simulink model "VCU_CS75_12_27_test"  (R2014a)
settings: Solver=FixedStepDiscrete  StartTime=0.0  StopTime=25  FixedStep=0.0005  RelTol=1e-3
undefined symbols (not defined in the file): D1, D2, D3, ecucoder_acal, ErrorSumMax1, ErrorSumMax2, ErrorSumMax3, I1, I2, I3, I_SW01_L, LaterlAngleCommand, LDW, P1, P2, P3, RemoteAcclPosition
libraries: simulink x913, ec5744lib x39
(part 12 of 30)

== system VCU_CS75_12_27_test/长安CS75底盘程序，20ms一次/Output/Subsystem/TransmitMessages5/ACC_3F5 ==
  ACC_AEBTargetLngRange_in : Inport
  ACC_AEBTargetRelSpeed_in : Inport  Port=2
  ACC_AEBTargetLatRange_in : Inport  Port=3
  ACC_HostPotentialTargetLatRng_in : Inport  Port=4
  ACC_HostPotentialTargetDetection_in : Inport  Port=5
  ACC_HostPotentialTargetLngRng_in : Inport  Port=6
  RollingConter_in : Inport  Port=7
  ACC_HostPotentialTargetType_in : Inport  Port=8
  CRC_in : Inport  Port=9
  ACC_3F5_DLC : Constant  Value=8  OutDataTypeStr=uint8
  ACC_3F5_DLC_Out : Terminator
  ACC_3F5_ID : Constant  Value=1013  OutDataTypeStr=single
  ACC_3F5_ID_Out : Terminator
  ACC_3F5_mux : Mux  Inputs=8
  ACC_AEBTargetLatRange : Subsystem
  ACC_AEBTargetLngRange : Subsystem
  ACC_AEBTargetRelSpeed : Subsystem
  ACC_HostPotentialTargetDetection : Subsystem
  ACC_HostPotentialTargetLatRng : Subsystem
  ACC_HostPotentialTargetLngRng : Subsystem
  ACC_HostPotentialTargetType : Subsystem
  CRC : Subsystem
  Conv{1..8} (8 alike) : DataTypeConversion
  RollingConter : Subsystem
  or{1..8} (8 alike) : simulink/Logic and Bit Operations/Bitwise Operator  logicop=OR  UseBitMask=off  NumInputPorts=9  BitMask=bin2dec('11011001')  BitMaskRealWorld=Stored Integer
  output : Outport
  wires:
  ACC_3F5_mux/1 -> output/1
  ACC_AEBTargetLngRange/1(output1) -> or1/1
  ACC_AEBTargetLngRange/2(output2) -> or2/1
  ACC_AEBTargetLngRange/3(output3) -> or3/1
  ACC_AEBTargetLngRange/4(output4) -> or4/1
  ACC_AEBTargetLngRange/5(output5) -> or5/1
  ACC_AEBTargetLngRange/6(output6) -> or6/1
  ACC_AEBTargetLngRange/7(output7) -> or7/1
  ACC_AEBTargetLngRange/8(output8) -> or8/1
  ACC_AEBTargetRelSpeed/1(output1) -> or1/2
  ACC_AEBTargetRelSpeed/2(output2) -> or2/2
  ACC_AEBTargetRelSpeed/3(output3) -> or3/2
  ACC_AEBTargetRelSpeed/4(output4) -> or4/2
  ACC_AEBTargetRelSpeed/5(output5) -> or5/2
  ACC_AEBTargetRelSpeed/6(output6) -> or6/2
  ACC_AEBTargetRelSpeed/7(output7) -> or7/2
  ACC_AEBTargetRelSpeed/8(output8) -> or8/2
  ACC_AEBTargetLatRange/1(output1) -> or1/3
  ACC_AEBTargetLatRange/2(output2) -> or2/3
  ACC_AEBTargetLatRange/3(output3) -> or3/3
  ACC_AEBTargetLatRange/4(output4) -> or4/3
  ACC_AEBTargetLatRange/5(output5) -> or5/3
  ACC_AEBTargetLatRange/6(output6) -> or6/3
  ACC_AEBTargetLatRange/7(output7) -> or7/3
  ACC_AEBTargetLatRange/8(output8) -> or8/3
  ACC_HostPotentialTargetLatRng/1(output1) -> or1/4
  ACC_HostPotentialTargetLatRng/2(output2) -> or2/4
  ACC_HostPotentialTargetLatRng/3(output3) -> or3/4
  ACC_HostPotentialTargetLatRng/4(output4) -> or4/4
  ACC_HostPotentialTargetLatRng/5(output5) -> or5/4
  ACC_HostPotentialTargetLatRng/6(output6) -> or6/4
  ACC_HostPotentialTargetLatRng/7(output7) -> or7/4
  ACC_HostPotentialTargetLatRng/8(output8) -> or8/4
  ACC_HostPotentialTargetDetection/1(output1) -> or1/5
  ACC_HostPotentialTargetDetection/2(output2) -> or2/5
  ACC_HostPotentialTargetDetection/3(output3) -> or3/5
  ACC_HostPotentialTargetDetection/4(output4) -> or4/5
  ACC_HostPotentialTargetDetection/5(output5) -> or5/5
  ACC_HostPotentialTargetDetection/6(output6) -> or6/5
  ACC_HostPotentialTargetDetection/7(output7) -> or7/5
  ACC_HostPotentialTargetDetection/8(output8) -> or8/5
  ACC_HostPotentialTargetLngRng/1(output1) -> or1/6
  ACC_HostPotentialTargetLngRng/2(output2) -> or2/6
  ACC_HostPotentialTargetLngRng/3(output3) -> or3/6
  ACC_HostPotentialTargetLngRng/4(output4) -> or4/6
  ACC_HostPotentialTargetLngRng/5(output5) -> or5/6
  ACC_HostPotentialTargetLngRng/6(output6) -> or6/6
  ACC_HostPotentialTargetLngRng/7(output7) -> or7/6
  ACC_HostPotentialTargetLngRng/8(output8) -> or8/6
  RollingConter/1(output1) -> or1/7
  RollingConter/2(output2) -> or2/7
  RollingConter/3(output3) -> or3/7
  RollingConter/4(output4) -> or4/7
  RollingConter/5(output5) -> or5/7
  RollingConter/6(output6) -> or6/7
  RollingConter/7(output7) -> or7/7
  RollingConter/8(output8) -> or8/7
  ACC_HostPotentialTargetType/1(output1) -> or1/8
  ACC_HostPotentialTargetType/2(output2) -> or2/8
  ACC_HostPotentialTargetType/3(output3) -> or3/8
  ACC_HostPotentialTargetType/4(output4) -> or4/8
  ACC_HostPotentialTargetType/5(output5) -> or5/8
  ACC_HostPotentialTargetType/6(output6) -> or6/8
  ACC_HostPotentialTargetType/7(output7) -> or7/8
  ACC_HostPotentialTargetType/8(output8) -> or8/8
  CRC/1(output1) -> or1/9
  CRC/2(output2) -> or2/9
  CRC/3(output3) -> or3/9
  CRC/4(output4) -> or4/9
  CRC/5(output5) -> or5/9
  CRC/6(output6) -> or6/9
  CRC/7(output7) -> or7/9
  CRC/8(output8) -> or8/9
  or1/1 -> Conv1/1
  Conv1/1 -> ACC_3F5_mux/1
  or2/1 -> Conv2/1
  Conv2/1 -> ACC_3F5_mux/2
  or3/1 -> Conv3/1
  Conv3/1 -> ACC_3F5_mux/3
  or4/1 -> Conv4/1
  Conv4/1 -> ACC_3F5_mux/4
  or5/1 -> Conv5/1
  Conv5/1 -> ACC_3F5_mux/5
  or6/1 -> Conv6/1
  Conv6/1 -> ACC_3F5_mux/6
  or7/1 -> Conv7/1
  Conv7/1 -> ACC_3F5_mux/7
  or8/1 -> Conv8/1
  Conv8/1 -> ACC_3F5_mux/8
  ACC_3F5_ID/1 -> ACC_3F5_ID_Out/1
  ACC_3F5_DLC/1 -> ACC_3F5_DLC_Out/1
  ACC_AEBTargetLngRange_in/1 -> ACC_AEBTargetLngRange/1(ACC_AEBTargetLngRange)
  ACC_AEBTargetRelSpeed_in/1 -> ACC_AEBTargetRelSpeed/1(ACC_AEBTargetRelSpeed)
  ACC_AEBTargetLatRange_in/1 -> ACC_AEBTargetLatRange/1(ACC_AEBTargetLatRange)
  ACC_HostPotentialTargetLatRng_in/1 -> ACC_HostPotentialTargetLatRng/1(ACC_HostPotentialTargetLatRng)
  ACC_HostPotentialTargetDetection_in/1 -> ACC_HostPotentialTargetDetection/1(ACC_HostPotentialTargetDetection)
  ACC_HostPotentialTargetLngRng_in/1 -> ACC_HostPotentialTargetLngRng/1(ACC_HostPotentialTargetLngRng)
  RollingConter_in/1 -> RollingConter/1(RollingConter)
  ACC_HostPotentialTargetType_in/1 -> ACC_HostPotentialTargetType/1(ACC_HostPotentialTargetType)
  CRC_in/1 -> CRC/1(CRC)

== system VCU_CS75_12_27_test/长安CS75底盘程序，20ms一次/Output/Subsystem/TransmitMessages7/APA_29A ==
  APA_EPBrequest_in : Inport
  APA_EPBrequestValid_in : Inport  Port=2
  APA_TranShiftReqValid_in : Inport  Port=3
  APA_TranShiftRequest_in : Inport  Port=4
  APA_TargetAcceleration_in : Inport  Port=5
  APA_TargetAccelerationValid_in : Inport  Port=6
  APA_GearReqValid_in : Inport  Port=7
  APA_LSCAction_in : Inport  Port=8
  APA_ActivationStatus_in : Inport  Port=9
  APA_RollingCounter_in : Inport  Port=10
  APA_Checksum_in : Inport  Port=11
  APA_29A_DLC : Constant  Value=8  OutDataTypeStr=uint8
  APA_29A_DLC_Out : Terminator
  APA_29A_ID : Constant  Value=666  OutDataTypeStr=single
  APA_29A_ID_Out : Terminator
  APA_29A_mux : Mux  Inputs=8
  APA_ActivationStatus : Subsystem
  APA_Checksum : Subsystem
  APA_EPBrequest : Subsystem
  APA_EPBrequestValid : Subsystem
  APA_GearReqValid : Subsystem
  APA_LSCAction : Subsystem
  APA_RollingCounter : Subsystem
  APA_TargetAcceleration : Subsystem
  APA_TargetAccelerationValid : Subsystem
  APA_TranShiftReqValid : Subsystem
  APA_TranShiftRequest : Subsystem
  Conv{1..8} (8 alike) : DataTypeConversion
  or{1..8} (8 alike) : simulink/Logic and Bit Operations/Bitwise Operator  logicop=OR  UseBitMask=off  NumInputPorts=11  BitMask=bin2dec('11011001')  BitMaskRealWorld=Stored Integer
  output : Outport
  wires:
  APA_29A_mux/1 -> output/1
  APA_EPBrequest/1(output1) -> or1/1
  APA_EPBrequest/2(output2) -> or2/1
  APA_EPBrequest/3(output3) -> or3/1
  APA_EPBrequest/4(output4) -> or4/1
  APA_EPBrequest/5(output5) -> or5/1
  APA_EPBrequest/6(output6) -> or6/1
  APA_EPBrequest/7(output7) -> or7/1
  APA_EPBrequest/8(output8) -> or8/1
  APA_EPBrequestValid/1(output1) -> or1/2
  APA_EPBrequestValid/2(output2) -> or2/2
  APA_EPBrequestValid/3(output3) -> or3/2
  APA_EPBrequestValid/4(output4) -> or4/2
  APA_EPBrequestValid/5(output5) -> or5/2
  APA_EPBrequestValid/6(output6) -> or6/2
  APA_EPBrequestValid/7(output7) -> or7/2
  APA_EPBrequestValid/8(output8) -> or8/2
  APA_TranShiftReqValid/1(output1) -> or1/3
  APA_TranShiftReqValid/2(output2) -> or2/3
  APA_TranShiftReqValid/3(output3) -> or3/3
  APA_TranShiftReqValid/4(output4) -> or4/3
  APA_TranShiftReqValid/5(output5) -> or5/3
  APA_TranShiftReqValid/6(output6) -> or6/3
  APA_TranShiftReqValid/7(output7) -> or7/3
  APA_TranShiftReqValid/8(output8) -> or8/3
  APA_TranShiftRequest/1(output1) -> or1/4
  APA_TranShiftRequest/2(output2) -> or2/4
  APA_TranShiftRequest/3(output3) -> or3/4
  APA_TranShiftRequest/4(output4) -> or4/4
  APA_TranShiftRequest/5(output5) -> or5/4
  APA_TranShiftRequest/6(output6) -> or6/4
  APA_TranShiftRequest/7(output7) -> or7/4
  APA_TranShiftRequest/8(output8) -> or8/4
  APA_TargetAcceleration/1(output1) -> or1/5
  APA_TargetAcceleration/2(output2) -> or2/5
  APA_TargetAcceleration/3(output3) -> or3/5
  APA_TargetAcceleration/4(output4) -> or4/5
  APA_TargetAcceleration/5(output5) -> or5/5
  APA_TargetAcceleration/6(output6) -> or6/5
  APA_TargetAcceleration/7(output7) -> or7/5
  APA_TargetAcceleration/8(output8) -> or8/5
  APA_TargetAccelerationValid/1(output1) -> or1/6
  APA_TargetAccelerationValid/2(output2) -> or2/6
  APA_TargetAccelerationValid/3(output3) -> or3/6
  APA_TargetAccelerationValid/4(output4) -> or4/6
  APA_TargetAccelerationValid/5(output5) -> or5/6
  APA_TargetAccelerationValid/6(output6) -> or6/6
  APA_TargetAccelerationValid/7(output7) -> or7/6
  APA_TargetAccelerationValid/8(output8) -> or8/6
  APA_GearReqValid/1(output1) -> or1/7
  APA_GearReqValid/2(output2) -> or2/7
  APA_GearReqValid/3(output3) -> or3/7
  APA_GearReqValid/4(output4) -> or4/7
  APA_GearReqValid/5(output5) -> or5/7
  APA_GearReqValid/6(output6) -> or6/7
  APA_GearReqValid/7(output7) -> or7/7
  APA_GearReqValid/8(output8) -> or8/7
  APA_LSCAction/1(output1) -> or1/8
  APA_LSCAction/2(output2) -> or2/8
  APA_LSCAction/3(output3) -> or3/8
  APA_LSCAction/4(output4) -> or4/8
  APA_LSCAction/5(output5) -> or5/8
  APA_LSCAction/6(output6) -> or6/8
  APA_LSCAction/7(output7) -> or7/8
  APA_LSCAction/8(output8) -> or8/8
  APA_ActivationStatus/1(output1) -> or1/9
  APA_ActivationStatus/2(output2) -> or2/9
  APA_ActivationStatus/3(output3) -> or3/9
  APA_ActivationStatus/4(output4) -> or4/9
  APA_ActivationStatus/5(output5) -> or5/9
  APA_ActivationStatus/6(output6) -> or6/9
  APA_ActivationStatus/7(output7) -> or7/9
  APA_ActivationStatus/8(output8) -> or8/9
  APA_RollingCounter/1(output1) -> or1/10
  APA_RollingCounter/2(output2) -> or2/10
  APA_RollingCounter/3(output3) -> or3/10
  APA_RollingCounter/4(output4) -> or4/10
  APA_RollingCounter/5(output5) -> or5/10
  APA_RollingCounter/6(output6) -> or6/10
  APA_RollingCounter/7(output7) -> or7/10
  APA_RollingCounter/8(output8) -> or8/10
  APA_Checksum/1(output1) -> or1/11
  APA_Checksum/2(output2) -> or2/11
  APA_Checksum/3(output3) -> or3/11
  APA_Checksum/4(output4) -> or4/11
  APA_Checksum/5(output5) -> or5/11
  APA_Checksum/6(output6) -> or6/11
  APA_Checksum/7(output7) -> or7/11
  APA_Checksum/8(output8) -> or8/11
  or1/1 -> Conv1/1
  Conv1/1 -> APA_29A_mux/1
  or2/1 -> Conv2/1
  Conv2/1 -> APA_29A_mux/2
  or3/1 -> Conv3/1
  Conv3/1 -> APA_29A_mux/3
  or4/1 -> Conv4/1
  Conv4/1 -> APA_29A_mux/4
  or5/1 -> Conv5/1
  Conv5/1 -> APA_29A_mux/5
  or6/1 -> Conv6/1
  Conv6/1 -> APA_29A_mux/6
  or7/1 -> Conv7/1
  Conv7/1 -> APA_29A_mux/7
  or8/1 -> Conv8/1
  Conv8/1 -> APA_29A_mux/8
  APA_29A_ID/1 -> APA_29A_ID_Out/1
  APA_29A_DLC/1 -> APA_29A_DLC_Out/1
  APA_EPBrequest_in/1 -> APA_EPBrequest/1(APA_EPBrequest)
  APA_EPBrequestValid_in/1 -> APA_EPBrequestValid/1(APA_EPBrequestValid)
  APA_TranShiftReqValid_in/1 -> APA_TranShiftReqValid/1(APA_TranShiftReqValid)
  APA_TranShiftRequest_in/1 -> APA_TranShiftRequest/1(APA_TranShiftRequest)
  APA_TargetAcceleration_in/1 -> APA_TargetAcceleration/1(APA_TargetAcceleration)
  APA_TargetAccelerationValid_in/1 -> APA_TargetAccelerationValid/1(APA_TargetAccelerationValid)
  APA_GearReqValid_in/1 -> APA_GearReqValid/1(APA_GearReqValid)
  APA_LSCAction_in/1 -> APA_LSCAction/1(APA_LSCAction)
  APA_ActivationStatus_in/1 -> APA_ActivationStatus/1(APA_ActivationStatus)
  APA_RollingCounter_in/1 -> APA_RollingCounter/1(APA_RollingCounter)
  APA_Checksum_in/1 -> APA_Checksum/1(APA_Checksum)

== system VCU_CS75_12_27_test/长安CS75底盘程序，20ms一次/Output/Subsystem/TransmitMessages8/APA_2D4 ==
  APA_APAStatus_in : Inport
  APA_ReleasePressureReq_in : Inport  Port=2
  RollingConter_in : Inport  Port=3
  CRC_in : Inport  Port=4
  APA_2D4_DLC : Constant  Value=8  OutDataTypeStr=uint8
  APA_2D4_DLC_Out : Terminator
  APA_2D4_ID : Constant  Value=724  OutDataTypeStr=single
  APA_2D4_ID_Out : Terminator
  APA_2D4_mux : Mux  Inputs=8
  APA_APAStatus : Subsystem
  APA_ReleasePressureReq : Subsystem
  CRC : Subsystem
  Conv{1..8} (8 alike) : DataTypeConversion
  RollingConter : Subsystem
  or{1..8} (8 alike) : simulink/Logic and Bit Operations/Bitwise Operator  logicop=OR  UseBitMask=off  NumInputPorts=4  BitMask=bin2dec('11011001')  BitMaskRealWorld=Stored Integer
  output : Outport
  wires:
  APA_2D4_mux/1 -> output/1
  APA_APAStatus/1(output1) -> or1/1
  APA_APAStatus/2(output2) -> or2/1
  APA_APAStatus/3(output3) -> or3/1
  APA_APAStatus/4(output4) -> or4/1
  APA_APAStatus/5(output5) -> or5/1
  APA_APAStatus/6(output6) -> or6/1
  APA_APAStatus/7(output7) -> or7/1
  APA_APAStatus/8(output8) -> or8/1
  APA_ReleasePressureReq/1(output1) -> or1/2
  APA_ReleasePressureReq/2(output2) -> or2/2
  APA_ReleasePressureReq/3(output3) -> or3/2
  APA_ReleasePressureReq/4(output4) -> or4/2
  APA_ReleasePressureReq/5(output5) -> or5/2
  APA_ReleasePressureReq/6(output6) -> or6/2
  APA_ReleasePressureReq/7(output7) -> or7/2
  APA_ReleasePressureReq/8(output8) -> or8/2
  RollingConter/1(output1) -> or1/3
  RollingConter/2(output2) -> or2/3
  RollingConter/3(output3) -> or3/3
  RollingConter/4(output4) -> or4/3
  RollingConter/5(output5) -> or5/3
  RollingConter/6(output6) -> or6/3
  RollingConter/7(output7) -> or7/3
  RollingConter/8(output8) -> or8/3
  CRC/1(output1) -> or1/4
  CRC/2(output2) -> or2/4
  CRC/3(output3) -> or3/4
  CRC/4(output4) -> or4/4
  CRC/5(output5) -> or5/4
  CRC/6(output6) -> or6/4
  CRC/7(output7) -> or7/4
  CRC/8(output8) -> or8/4
  or1/1 -> Conv1/1
  Conv1/1 -> APA_2D4_mux/1
  or2/1 -> Conv2/1
  Conv2/1 -> APA_2D4_mux/2
  or3/1 -> Conv3/1
  Conv3/1 -> APA_2D4_mux/3
  or4/1 -> Conv4/1
  Conv4/1 -> APA_2D4_mux/4
  or5/1 -> Conv5/1
  Conv5/1 -> APA_2D4_mux/5
  or6/1 -> Conv6/1
  Conv6/1 -> APA_2D4_mux/6
  or7/1 -> Conv7/1
  Conv7/1 -> APA_2D4_mux/7
  or8/1 -> Conv8/1
  Conv8/1 -> APA_2D4_mux/8
  APA_2D4_ID/1 -> APA_2D4_ID_Out/1
  APA_2D4_DLC/1 -> APA_2D4_DLC_Out/1
  APA_APAStatus_in/1 -> APA_APAStatus/1(APA_APAStatus)
  APA_ReleasePressureReq_in/1 -> APA_ReleasePressureReq/1(APA_ReleasePressureReq)
  RollingConter_in/1 -> RollingConter/1(RollingConter)
  CRC_in/1 -> CRC/1(CRC)

== system VCU_CS75_12_27_test/长安CS75底盘程序，20ms一次/Input/CAN0_Rx/a1_211/ReceiveMessages/Subsystem ==
  note: -5~100
  note: -100~100
  input : Inport
  Enable : EnablePort
  Bus Creator : BusCreator  Inputs=5
  Constant : Constant  Value=0  SampleTime=-1
  Constant1 : Constant  Value=0  SampleTime=-1
  Constant2 : Constant  Value=0  SampleTime=-1
  Data Store Write : DataStoreWrite  DataStoreName=Vx_out  DataStoreElements=Vx_out
  Data Store Write1 : DataStoreWrite  DataStoreName=mission_out  DataStoreElements=mission_out
  Data Store Write2 : DataStoreWrite  DataStoreName=SCS_out  DataStoreElements=SCS_out
  Data Store Write3 : DataStoreWrite  DataStoreName=finish_out  DataStoreElements=finish_out
  Data Store Write4 : DataStoreWrite  DataStoreName=tap_out  DataStoreElements=tap_out
  Data Store Write5 : DataStoreWrite  DataStoreName=cones_count_all_out  DataStoreElements=cones_count_all_out
  Data Store Write6 : DataStoreWrite  DataStoreName=cones_count_actual_out  DataStoreElements=cones_count_actual_out
  Data Type Conversion : DataTypeConversion  OutDataTypeStr=double
  MATLAB Function1 : MATLAB Function  TreatAsAtomicUnit=on
  Signal Conversion : SignalConversion
  a1 : Subsystem
  A1_211 : Outport
  wires:
  MATLAB Function1/1(y) -> Bus Creator/2  "RemoteAcclPosition"
  Constant/1 -> Bus Creator/4  "A1_Message_Counter"
  Constant1/1 -> Bus Creator/5  "A1_Checksum"
  input/1 -> a1/1(input)
  Constant2/1 -> Bus Creator/1  "AutoDrivingReady"
  a1/8(throttlevbrake_position_Out) -> Data Type Conversion/1  "RemoteAcclPosition"
  a1/1(Vx_Out) -> Data Store Write/1
  a1/2(mission_Out) -> Data Store Write1/1
  a1/3(SCS_Out) -> Data Store Write2/1
  a1/4(finish_Out) -> Data Store Write3/1
  a1/5(tap_Out) -> Data Store Write4/1
  a1/6(cones_count_all_Out) -> Data Store Write5/1
  a1/7(cones_count_actual_Out) -> Data Store Write6/1
  Bus Creator/1 -> Signal Conversion/1
  Data Type Conversion/1 -> MATLAB Function1/1(u)
  Signal Conversion/1 -> A1_211/1
  a1/9(target_steering_Out) -> Bus Creator/3  "LaterlAngleCommand"

== system VCU_CS75_12_27_test/长安CS75底盘程序，20ms一次/Input/CAN1_Rx/BCM_288/ReceiveMessages/Subsystem ==
  input : Inport
  Enable : EnablePort
  BCM_1 : Subsystem
  Bus Creator : BusCreator  Inputs=20
  Signal Conversion : SignalConversion
  BCM_288 : Outport
  wires:
  Bus Creator/1 -> Signal Conversion/1
  input/1 -> BCM_1/1(input)
  BCM_1/1(BCM_FrontWashStatus_Out) -> Bus Creator/1  "BCM_FrontWashStatus"
  BCM_1/2(BCM_TurnIndicatorRight_Out) -> Bus Creator/2  "BCM_TurnIndicatorRight"
  BCM_1/3(BCM_TurnIndicatorLeft_Out) -> Bus Creator/3  "BCM_TurnIndicatorLeft"
  BCM_1/4(BCM_HoodStatus_Out) -> Bus Creator/4  "BCM_HoodStatus"
  BCM_1/5(BCM_TrunkDoorStatus_Out) -> Bus Creator/5  "BCM_TrunkDoorStatus"
  BCM_1/6(BCM_RightRearDoorStatus_Out) -> Bus Creator/6  "BCM_RightRearDoorStatus"
  BCM_1/7(BCM_LeftRearDoorStatus_Out) -> Bus Creator/7  "BCM_LeftRearDoorStatus"
  BCM_1/8(BCM_PassengerDoorStatus_Out) -> Bus Creator/8  "BCM_PassengerDoorStatus"
  BCM_1/9(BCM_DriverDoorStatus_Out) -> Bus Creator/9  "BCM_DriverDoorStatus"
  BCM_1/10(BCM_PassengerDoorLockStatus_Out) -> Bus Creator/10  "BCM_PassengerDoorLockStatus"
  BCM_1/11(BCM_emergencylightstatus_Out) -> Bus Creator/11  "BCM_emergencylightstatus"
  BCM_1/12(BCM_DriverDoorLockStatus_Out) -> Bus Creator/12  "BCM_DriverDoorLockStatus"
  BCM_1/13(BCM_PowerStatusFeedback_Out) -> Bus Creator/13  "BCM_PowerStatusFeedback"
  BCM_1/14(BCM_RearWiperStatus_Out) -> Bus Creator/14  "BCM_RearWiperStatus"
  BCM_1/15(BCM_FrontWiperStatus_Out) -> Bus Creator/15  "BCM_FrontWiperStatus"
  BCM_1/16(BCM_ReversePosition_Out) -> Bus Creator/16  "BCM_ReversePosition"
  BCM_1/17(BCM_TurnLightSwitchSts_Out) -> Bus Creator/17  "BCM_TurnLightSwitchSts"
  BCM_1/18(BCM_BuzzerWarningMode_Out) -> Bus Creator/18  "BCM_BuzzerWarningMode"
  BCM_1/19(BCM_SystemFailureFlag_Out) -> Bus Creator/19  "BCM_SystemFailureFlag"
  BCM_1/20(BCM_LatchOverheatProtect_Out) -> Bus Creator/20  "BCM_LatchOverheatProtect"
  Signal Conversion/1 -> BCM_288/1

== system VCU_CS75_12_27_test/长安CS75底盘程序，20ms一次/Input/CAN1_Rx/BCM_328/ReceiveMessages/Subsystem ==
  input : Inport
  Enable : EnablePort
  BCM_1 : Subsystem
  Bus Creator : BusCreator  Inputs=6
  Signal Conversion : SignalConversion
  BCM_328 : Outport
  wires:
  Bus Creator/1 -> Signal Conversion/1
  input/1 -> BCM_1/1(input)
  BCM_1/1(LCM_DriveMode_Out) -> Bus Creator/1  "LCM_DriveMode"
  BCM_1/2(LCM_DRLSts_Out) -> Bus Creator/2  "LCM_DRLSts"
  BCM_1/3(LCM_LASSwitch_Out) -> Bus Creator/3  "LCM_LASSwitch"
  BCM_1/4(LCM_RearRightTuningLightFaultSts_Out) -> Bus Creator/4  "LCM_RearRightTuningLightFaultSts"
  BCM_1/5(LCM_RearLeftTuningLightFaultSts_Out) -> Bus Creator/5  "LCM_RearLeftTuningLightFaultSts"
  BCM_1/6(LCM_ReverseLightSts_Out) -> Bus Creator/6  "LCM_ReverseLightSts"
  Signal Conversion/1 -> BCM_328/1

== system VCU_CS75_12_27_test/长安CS75底盘程序，20ms一次/Input/CAN1_Rx/BCM_348/ReceiveMessages/Subsystem ==
  input : Inport
  Enable : EnablePort
  BCM_1 : Subsystem
  Bus Creator : BusCreator  Inputs=3
  Signal Conversion : SignalConversion
  BCM_348 : Outport
  wires:
  input/1 -> BCM_1/1(input)
  Bus Creator/1 -> Signal Conversion/1
  BCM_1/1(BCM_DriveMode_Out) -> Bus Creator/1  "BCM_DriveMode"
  BCM_1/2(BCM_LockSignal_Out) -> Bus Creator/2  "BCM_LockSignal"
  BCM_1/3(BCM_UnlockSignal_Out) -> Bus Creator/3  "BCM_UnlockSignal"
  Signal Conversion/1 -> BCM_348/1

== system VCU_CS75_12_27_test/长安CS75底盘程序，20ms一次/Input/CAN1_Rx/BCM_3DF/ReceiveMessages/Subsystem ==
  input : Inport
  Enable : EnablePort
  BCM_3DF1 : Subsystem
  Bus Creator : BusCreator  Inputs=8
  Signal Conversion : SignalConversion
  BCM_3DF : Outport
  wires:
  Bus Creator/1 -> Signal Conversion/1
  input/1 -> BCM_3DF1/1(input)
  BCM_3DF1/1(BCM_DriveMode_Out) -> Bus Creator/1  "BCM_DriveMode"
  BCM_3DF1/2(BCM_EPSTorqueMode_Out) -> Bus Creator/2  "BCM_EPSTorqueMode"
  BCM_3DF1/3(BCM_DriveModeStatus_Out) -> Bus Creator/3  "BCM_DriveModeStatus"
  BCM_3DF1/4(BCM_DriveModeFeedback_Out) -> Bus Creator/4  "BCM_DriveModeFeedback"
  BCM_3DF1/5(BCM_EPSTorqueModeFeedback_Out) -> Bus Creator/5  "BCM_EPSTorqueModeFeedback"
  BCM_3DF1/6(BCM_AmbientLightColorFeedback_Out) -> Bus Creator/6  "BCM_AmbientLightColorFeedback"
  BCM_3DF1/7(BCM_RollingCounter_Out) -> Bus Creator/7  "BCM_RollingCounter"
  BCM_3DF1/8(BCM_CRC_Checksum_Out) -> Bus Creator/8  "BCM_CRC_Checksum"
  Signal Conversion/1 -> BCM_3DF/1

== system VCU_CS75_12_27_test/长安CS75底盘程序，20ms一次/Input/CAN1_Rx/EMS_205/ReceiveMessages/Subsystem ==
  input : Inport
  Enable : EnablePort
  Bus Creator : BusCreator  Inputs=7
  EMS : Subsystem
  Signal Conversion : SignalConversion
  EMS_205 : Outport
  wires:
  EMS/1(EMS_ESPTorqReuestAvailability_Out) -> Bus Creator/1  "EMS_ESPTorqReuestAvailability"
  EMS/2(EMS_TorqFailure_Out) -> Bus Creator/2  "EMS_TorqFailure"
  EMS/3(EMS_IndicatedDriverReqTorq_Out) -> Bus Creator/3  "EMS_IndicatedDriverReqTorq"
  EMS/4(EMS_FrictionalTorq_Out) -> Bus Creator/4  "EMS_FrictionalTorq"
  EMS/5(EMS_IndicatedRealEngTorq_Out) -> Bus Creator/5  "EMS_IndicatedRealEngTorq"
  EMS/6(EMS_RollingCounter_id205_Out) -> Bus Creator/6  "EMS_RollingCounter_id205"
  EMS/7(EMS_CheckSum_205_Out) -> Bus Creator/7  "EMS_CheckSum_205"
  input/1 -> EMS/1(input)
  Bus Creator/1 -> Signal Conversion/1
  Signal Conversion/1 -> EMS_205/1

== system VCU_CS75_12_27_test/长安CS75底盘程序，20ms一次/Input/CAN1_Rx/EMS_255/ReceiveMessages/Subsystem ==
  input : Inport
  Enable : EnablePort
  Bus Creator : BusCreator  Inputs=7
  EMS : Subsystem
  Signal Conversion : SignalConversion
  EMS_255 : Outport
  wires:
  input/1 -> EMS/1(input)
  Bus Creator/1 -> Signal Conversion/1
  EMS/1(EMS_BrakePedalStatus_Out) -> Bus Creator/1  "EMS_BrakePedalStatus"
  EMS/2(EMS_AccpedelError_Out) -> Bus Creator/2  "EMS_AccpedelError"
  EMS/3(EMS_EngineSpeedError_Out) -> Bus Creator/3  "EMS_EngineSpeedError"
  EMS/4(EMS_EngineSpeed_Out) -> Bus Creator/4  "EMS_EngineSpeed"
  EMS/5(EMS_AccPedal_Out) -> Bus Creator/5  "EMS_AccPedal"
  EMS/6(EMS_RollingCounter_id255_Out) -> Bus Creator/6  "EMS_RollingCounter_id255"
  EMS/7(EMS_CheckSum_255_Out) -> Bus Creator/7  "EMS_CheckSum_255"
  Signal Conversion/1 -> EMS_255/1

== system VCU_CS75_12_27_test/长安CS75底盘程序，20ms一次/Input/CAN1_Rx/EMS_265/ReceiveMessages/Subsystem ==
  input : Inport
  Enable : EnablePort
  Bus Creator : BusCreator
  EMS_265xx : Subsystem
  Signal Conversion : SignalConversion
  EMS_265 : Outport
  wires:
  EMS_265xx/4(EMS_EngineStatus_Out) -> Bus Creator/4  "EMS_EngineStatus"
  EMS_265xx/3(EMS_RollingCounter_id265_Out) -> Bus Creator/3  "EMS_RollingCounter_id265"
  EMS_265xx/2(EMS_TorqueConstant_Out) -> Bus Creator/2  "EMS_TorqueConstant"
  EMS_265xx/1(EMS_FullLoadIndicatedTorq_Out) -> Bus Creator/1  "EMS_FullLoadIndicatedTorq"
  Bus Creator/1 -> Signal Conversion/1
  input/1 -> EMS_265xx/1(input)
  Signal Conversion/1 -> EMS_265/1

== system VCU_CS75_12_27_test/长安CS75底盘程序，20ms一次/Input/CAN1_Rx/EMS_276/ReceiveMessages/Subsystem ==
  input : Inport
  Enable : EnablePort
  Bus Creator : BusCreator  Inputs=1
  EMS_2 : Subsystem
  Signal Conversion : SignalConversion
  EMS_276 : Outport
  wires:
  input/1 -> EMS_2/1(input)
  Bus Creator/1 -> Signal Conversion/1
  EMS_2/1(EMS_RealAccPedal_Out) -> Bus Creator/1  "EMS_RealAccPedal"
  Signal Conversion/1 -> EMS_276/1

== system VCU_CS75_12_27_test/长安CS75底盘程序，20ms一次/Input/CAN1_Rx/EPB_256/ReceiveMessages/Subsystem ==
  input : Inport
  Enable : EnablePort
  Bus Creator : BusCreator  Inputs=6
  EPB : Subsystem
  Signal Conversion : SignalConversion
  EPB_256 : Outport
  wires:
  EPB/1(EPB_FailStatus_Out) -> Bus Creator/1  "EPB_FailStatus"
  Bus Creator/1 -> Signal Conversion/1
  input/1 -> EPB/1(input)
  EPB/2(EPB_Status_Out) -> Bus Creator/2  "EPB_Status"
  EPB/3(EPB_FunctionLamp_Out) -> Bus Creator/3  "EPB_FunctionLamp"
  EPB/4(EPB_FailureLamp_Out) -> Bus Creator/4  "EPB_FailureLamp"
  EPB/5(EPB_RollingCounter_id256_Out) -> Bus Creator/5  "EPB_RollingCounter_id256"
  EPB/6(EPB_Checksum_Out) -> Bus Creator/6  "EPB_Checksum"
  Signal Conversion/1 -> EPB_256/1

== system VCU_CS75_12_27_test/长安CS75底盘程序，20ms一次/Input/CAN1_Rx/EPS_20A/ReceiveMessages/Subsystem ==
  input : Inport
  Enable : EnablePort
  Bus Creator : BusCreator  Inputs=9
  EPS_20A1 : Subsystem
  Signal Conversion : SignalConversion
  EPS_20A : Outport
  wires:
  input/1 -> EPS_20A1/1(input)
  Bus Creator/1 -> Signal Conversion/1
  EPS_20A1/1(EPS_EPSFailed_Out) -> Bus Creator/1  "EPS_EPSFailed"
  EPS_20A1/2(EPS_APA_EpasFailed_Out) -> Bus Creator/2  "EPS_APA_EpasFailed"
  EPS_20A1/3(EPS_APA_AbortFeedback_Out) -> Bus Creator/3  "EPS_APA_AbortFeedback"
  EPS_20A1/4(EPS_SteeringTorque_Out) -> Bus Creator/4  "EPS_SteeringTorque"
  EPS_20A1/5(EPS_TorqueSensorStatus_Out) -> Bus Creator/5  "EPS_TorqueSensorStatus"
  EPS_20A1/6(EPS_APA_ControlFeedback_Out) -> Bus Creator/6  "EPS_APA_ControlFeedback"
  EPS_20A1/7(EPS_RollingCounter_Out) -> Bus Creator/7  "EPS_RollingCounter"
  EPS_20A1/8(EPS_ConcussAvailabilityStatus_Out) -> Bus Creator/8  "EPS_ConcussAvailabilityStatus"
  EPS_20A1/9(EPS_Checksum_Out) -> Bus Creator/9  "EPS_Checksum"
  Signal Conversion/1 -> EPS_20A/1

== system VCU_CS75_12_27_test/长安CS75底盘程序，20ms一次/Input/CAN1_Rx/EPS_21A/ReceiveMessages/Subsystem ==
  input : Inport
  Enable : EnablePort
  Bus Creator : BusCreator  Inputs=6
  EPS_21A2 : Subsystem
  Signal Conversion : SignalConversion
  EPS_21A : Outport
  wires:
  Bus Creator/1 -> Signal Conversion/1
  input/1 -> EPS_21A2/1(input)
  EPS_21A2/1(EPS_MeasuredTosionBatTorque_Out) -> Bus Creator/1  "EPS_MeasuredTosionBatTorque"
  EPS_21A2/2(EPS_AvailabilityStatus_Out) -> Bus Creator/2  "EPS_AvailabilityStatus"
  EPS_21A2/3(EPS_MeasTsionBatTorquevalid_Out) -> Bus Creator/3  "EPS_MeasTsionBatTorquevalid"
  EPS_21A2/4(EPS_IACC_abortReson_Out) -> Bus Creator/4  "EPS_IACC_abortReson"
  EPS_21A2/5(Rollingcounter_Out) -> Bus Creator/5  "EPS_21A_Rollingcounter"
  EPS_21A2/6(CRC_Out) -> Bus Creator/6  "EPS_21A_CheckingSum"
  Signal Conversion/1 -> EPS_21A/1

== system VCU_CS75_12_27_test/长安CS75底盘程序，20ms一次/Input/CAN1_Rx/ESP_277/ReceiveMessages/Subsystem ==
  input : Inport
  Enable : EnablePort
  Bus Creator : BusCreator  Inputs=19
  ESP_1 : Subsystem
  Signal Conversion : SignalConversion
  ESP_277 : Outport
  wires:
  Bus Creator/1 -> Signal Conversion/1
  input/1 -> ESP_1/1(input)
  ESP_1/1(ESP_BrakeForce_Out) -> Bus Creator/1  "ESP_BrakeForce"
  ESP_1/2(ESP_VDCActive_Out) -> Bus Creator/2  "ESP_VDCActive"
  ESP_1/3(ESP_TCSActive_Out) -> Bus Creator/3  "ESP_TCSActive"
  ESP_1/4(ESP_AWBavailable_Out) -> Bus Creator/4  "ESP_AWBavailable"
  ESP_1/5(ESP_AWBactive_Out) -> Bus Creator/5  "ESP_AWBactive"
  ESP_1/6(ESP_AEBdecActive_Out) -> Bus Creator/6  "ESP_AEBdecActive"
  ESP_1/7(ESP_AEBAvailable_Out) -> Bus Creator/7  "ESP_AEBAvailable"
  ESP_1/8(ESP_ABAavailable_Out) -> Bus Creator/8  "ESP_ABAavailable"
  ESP_1/9(ESP_ABAactive_Out) -> Bus Creator/9  "ESP_ABAactive"
  ESP_1/10(ESP_PrefillAvailable_Out) -> Bus Creator/10  "ESP_PrefillAvailable"
  ESP_1/11(ESP_PrefillActive_Out) -> Bus Creator/11  "ESP_PrefillActive"
  ESP_1/12(ESP_BrakeOverHeat_Out) -> Bus Creator/12  "ESP_BrakeOverHeat"
  ESP_1/13(ESP_CDD_Active_Out) -> Bus Creator/13  "ESP_CDD_Active"
  ESP_1/14(ESP_CDD_Available_Out) -> Bus Creator/14  "ESP_CDD_Available"
  ESP_1/15(ESP_CDD_Active_APA_Out) -> Bus Creator/15  "ESP_CDD_Active_APA"
  ESP_1/16(ESP_VehicleStandstill_Out) -> Bus Creator/16  "ESP_VehicleStandstill"
  ESP_1/17(ESP_CDD_Available_APA_Out) -> Bus Creator/17  "ESP_CDD_Available_APA"
  ESP_1/18(ESP_RollingCounter_277_Out) -> Bus Creator/18  "ESP_RollingCounter_277"
  ESP_1/19(ESP_CheckSum_277_Out) -> Bus Creator/19  "ESP_CheckSum_277"
  Signal Conversion/1 -> ESP_277/1

== system VCU_CS75_12_27_test/长安CS75底盘程序，20ms一次/Input/CAN1_Rx/ESP_280/ReceiveMessages/Subsystem ==
  input : Inport
  Enable : EnablePort
  Bus Creator : BusCreator  Inputs=12
  ESP_1 : Subsystem
  Signal Conversion : SignalConversion
  ESP_280 : Outport
  wires:
  input/1 -> ESP_1/1(input)
  Bus Creator/1 -> Signal Conversion/1
  ESP_1/12(Wheel_Speed_FL_Valid_Data_Out) -> Bus Creator/12  "Wheel_Speed_FL_Valid"
  ESP_1/11(Wheel_Speed_FL_Direction_Out) -> Bus Creator/11  "Wheel_Speed_FL_Direction"
  ESP_1/10(Wheel_Speed_FL_Data_Out) -> Bus Creator/10  "Wheel_Speed_FL"
  ESP_1/1(Wheel_Speed_RR_Data_Out) -> Bus Creator/1  "Wheel_Speed_RR"
  ESP_1/2(Wheel_Speed_RR_Direction_Out) -> Bus Creator/2  "Wheel_Speed_RR_Direction"
  ESP_1/3(Wheel_Speed_RR_Valid_Data_Out) -> Bus Creator/3  "Wheel_Speed_RR_Valid"
  ESP_1/4(Wheel_Speed_RL_Data_Out) -> Bus Creator/4  "Wheel_Speed_RL"
  ESP_1/5(Wheel_Speed_RL_Direction_Out) -> Bus Creator/5  "Wheel_Speed_RL_Direction"
  ESP_1/6(Wheel_Speed_RL_Valid_Data_Out) -> Bus Creator/6  "Wheel_Speed_RL_Valid"
  ESP_1/7(Wheel_Speed_FR_Data_Out) -> Bus Creator/7  "Wheel_Speed_FR"
  ESP_1/8(Wheel_Speed_FR_Direction_Out) -> Bus Creator/8  "Wheel_Speed_FR_Direction"
  ESP_1/9(Wheel_Speed_FR_Valid_Data_Out) -> Bus Creator/9  "Wheel_Speed_FR_Valid"
  Signal Conversion/1 -> ESP_280/1

== system VCU_CS75_12_27_test/长安CS75底盘程序，20ms一次/Input/CAN1_Rx/ESP_281/ReceiveMessages/Subsystem ==
  input : Inport
  Enable : EnablePort
  Bus Creator : BusCreator  Inputs=11
  ESP_2 : Subsystem
  Signal Conversion : SignalConversion
  ESP_281 : Outport
  wires:
  Bus Creator/1 -> Signal Conversion/1
  input/1 -> ESP_2/1(input)
  ESP_2/1(ESP_ESPActiveStatus_Out) -> Bus Creator/1  "ESP_ESPActiveStatus"
  ESP_2/2(ESP_ESPSwitchStatus_Out) -> Bus Creator/2  "ESP_ESPSwitchStatus"
  ESP_2/3(ESP_EBDFailStatus_Out) -> Bus Creator/3  "ESP_EBDFailStatus"
  ESP_2/4(ESP_ABSFailStatus_Out) -> Bus Creator/4  "ESP_ABSFailStatus"
  ESP_2/5(ESP_ESPFailStatus_Out) -> Bus Creator/5  "ESP_ESPFailStatus"
  ESP_2/6(ESP_ABSActiveStatus_Out) -> Bus Creator/6  "ESP_ABSActiveStatus"
  ESP_2/7(ESP_VehicleSpeed_Out) -> Bus Creator/7  "ESP_VehicleSpeed"
  ESP_2/8(ESP_VehicleSpeed_Status_Out) -> Bus Creator/8  "ESP_VehicleSpeed_Status"
  ESP_2/9(ESP_RollingCounter_Out) -> Bus Creator/9  "ESP_RollingCounter"
  ESP_2/10(ESP_BrakePedalStatus_Out) -> Bus Creator/10  "ESP_BrakePedalStatus"
  ESP_2/11(ESP_Checksum_Out) -> Bus Creator/11  "ESP_Checksum"
  Signal Conversion/1 -> ESP_281/1

== system VCU_CS75_12_27_test/长安CS75底盘程序，20ms一次/Input/CAN1_Rx/ESP_287/ReceiveMessages/Subsystem ==
  input : Inport
  Enable : EnablePort
  Bus Creator : BusCreator  Inputs=13
  ESP_2 : Subsystem
  Signal Conversion : SignalConversion
  ESP_287 : Outport
  wires:
  input/1 -> ESP_2/1(input)
  Bus Creator/1 -> Signal Conversion/1
  ESP_2/13(ESP_RollingCounter_Out) -> Bus Creator/13  "ESP_RollingCounter"
  ESP_2/12(ESP_CheckSum_Out) -> Bus Creator/12  "ESP_CheckSum"
  ESP_2/11(ESP_YawRate_Status_Out) -> Bus Creator/11  "ESP_YawRate_Status"
  ESP_2/10(ESP_LongAccelValid_Out) -> Bus Creator/10  "ESP_LongAccelValid"
  ESP_2/9(ESP_HBBActiveStatus_Out) -> Bus Creator/9  "ESP_HBBActiveStatus"
  ESP_2/8(ESP_HHC_Available_Out) -> Bus Creator/8  "ESP_HHC_Available"
  ESP_2/7(ESP_HBB_Status_Out) -> Bus Creator/7  "ESP_HBB_Status"
  ESP_2/6(ESP_YawRate_Out) -> Bus Creator/6  "ESP_YawRate"
  ESP_2/5(ESP_LongAcceleration_Out) -> Bus Creator/5  "ESP_LongAcceleration"
  ESP_2/4(ESP_LatAcceleration_Out) -> Bus Creator/4  "ESP_LatAcceleration"
  ESP_2/3(ESP_TODFastOpenRequest_Out) -> Bus Creator/3  "ESP_TODFastOpenRequest"
  ESP_2/2(ESP_HDC_Status_Out) -> Bus Creator/2  "ESP_HDC_Status"
  ESP_2/1(ESP_TODTorqueMaxLimit_Out) -> Bus Creator/1  "ESP_TODTorqueMaxLimit"
  Signal Conversion/1 -> ESP_287/1

== system VCU_CS75_12_27_test/长安CS75底盘程序，20ms一次/Input/CAN1_Rx/GW_20B/ReceiveMessages/Subsystem ==
  input : Inport
  Enable : EnablePort
  Bus Creator : BusCreator  Inputs=9
  GW_20B2 : Subsystem
  Signal Conversion : SignalConversion
  GW_20B : Outport
  wires:
  input/1 -> GW_20B2/1(input)
  Bus Creator/1 -> Signal Conversion/1
  GW_20B2/1(SAS_SteeringAngleValid_Out) -> Bus Creator/1  "SAS_SteeringAngleValid"
  GW_20B2/2(EMS_EngineStatus_Out) -> Bus Creator/2  "EMS_EngineStatus"
  GW_20B2/3(EMS_BrakePedalStatus_Out) -> Bus Creator/3  "EMS_BrakePedalStatus"
  GW_20B2/4(EMS_EngineStartupEnd_Out) -> Bus Creator/4  "EMS_EngineStartupEnd"
  GW_20B2/5(SAS_SteeringAngle_Out) -> Bus Creator/5  "SAS_SteeringAngle"
  GW_20B2/6(EPB_BrakeLightOnRequest_Out) -> Bus Creator/6  "EPB_BrakeLightOnRequest"
  GW_20B2/7(TCU_GearShiftPositon_Out) -> Bus Creator/7  "TCU_GearShiftPositon"
  GW_20B2/8(TCU_ShiftPostionValid_Out) -> Bus Creator/8  "TCU_ShiftPostionValid"
  GW_20B2/9(EPB_Status_Out) -> Bus Creator/9  "EPB_Status"
  Signal Conversion/1 -> GW_20B/1

== system VCU_CS75_12_27_test/长安CS75底盘程序，20ms一次/Input/CAN1_Rx/GW_308/ReceiveMessages/Subsystem ==
  input : Inport
  Enable : EnablePort
  Bus Creator : BusCreator  Inputs=1
  GW_1 : Subsystem
  Signal Conversion : SignalConversion
  GW_308 : Outport
  wires:
  input/1 -> GW_1/1(input)
  Bus Creator/1 -> Signal Conversion/1
  GW_1/1(IP_TotalOdometer_Out) -> Bus Creator/1  "IP_TotalOdometer"
  Signal Conversion/1 -> GW_308/1

== system VCU_CS75_12_27_test/长安CS75底盘程序，20ms一次/Input/CAN1_Rx/GW_332/ReceiveMessages/Subsystem ==
  input : Inport
  Enable : EnablePort
  Bus Creator : BusCreator
  GW_1 : Subsystem
  Signal Conversion : SignalConversion
  GW_332 : Outport
  wires:
  Bus Creator/1 -> Signal Conversion/1
  input/1 -> GW_1/1(input)
  GW_1/1(SRS_PassengerBuckleSwitchStatus_Out) -> Bus Creator/1  "SRS_PassengerBuckleSwitchStatus"
  GW_1/2(SRS_DriverBuckleSwitchStatus_Out) -> Bus Creator/2  "SRS_DriverBuckleSwitchStatus"
  GW_1/3(SAS_SASFailure_Out) -> Bus Creator/3  "SAS_SASFailure"
  GW_1/4(EMS_EngineSpeed_Out) -> Bus Creator/4  "EMS_EngineSpeed"
  Signal Conversion/1 -> GW_332/1

== system VCU_CS75_12_27_test/长安CS75底盘程序，20ms一次/Input/CAN1_Rx/GW_376/ReceiveMessages/Subsystem ==
  input : Inport
  Enable : EnablePort
  Bus Creator : BusCreator
  GW_2 : Subsystem
  Signal Conversion : SignalConversion
  GW_376 : Outport
  wires:
  Bus Creator/1 -> Signal Conversion/1
  input/1 -> GW_2/1(input)
  GW_2/1(EMS_TorqueConstant_Out) -> Bus Creator/1  "EMS_TorqueConstant"
  GW_2/2(EMS_FrictionalTorq_Out) -> Bus Creator/2  "EMS_FrictionalTorq"
  GW_2/3(EMS_EngineFuelCutOff_Out) -> Bus Creator/3  "EMS_EngineFuelCutOff"
  GW_2/4(EMS_ConditionIdle_Out) -> Bus Creator/4  "EMS_ConditionIdle"
  Signal Conversion/1 -> GW_376/1

== system VCU_CS75_12_27_test/长安CS75底盘程序，20ms一次/Input/CAN1_Rx/GW_3A2/ReceiveMessages/Subsystem ==
  input : Inport
  Enable : EnablePort
  Bus Creator : BusCreator  Inputs=27
  GW_3A1 : Subsystem
  Signal Conversion : SignalConversion
  GW_3A2 : Outport
  wires:
  input/1 -> GW_3A1/1(input)
  Bus Creator/1 -> Signal Conversion/1
  GW_3A1/1(EPS_TorqueAssistMode_Out) -> Bus Creator/1  "EPS_TorqueAssistMode"
  GW_3A1/2(EMS_RemindGear_Out) -> Bus Creator/2  "EMS_RemindGear"
  GW_3A1/3(TCU_FailureLamp_Out) -> Bus Creator/3  "TCU_FailureLamp"
  GW_3A1/4(ACC_ACCMode_Out) -> Bus Creator/4  "ACC_ACCMode"
  GW_3A1/5(TCU_WNTLamp_Out) -> Bus Creator/5  "TCU_WNTLamp"
  GW_3A1/6(TCU_PWRLamp_Out) -> Bus Creator/6  "TCU_PWRLamp"
  GW_3A1/7(SRS_LeftRearBuckleSwitchSts_Out) -> Bus Creator/7  "SRS_LeftRearBuckleSwitchSts"
  GW_3A1/8(SRS_MiddleRearBuckleSwitchSts_Out) -> Bus Creator/8  "SRS_MiddleRearBuckleSwitchSts"
  GW_3A1/9(SRS_RightRearBuckleSwitchSts_Out) -> Bus Creator/9  "SRS_RightRearBuckleSwitchSts"
  GW_3A1/10(EPB_TextDisplay_Out) -> Bus Creator/10  "EPB_TextDisplay"
  GW_3A1/11(ESP_ESPActiveStatus_Out) -> Bus Creator/11  "ESP_ESPActiveStatus"
  GW_3A1/12(ESP_ESPFunctionStatus_Out) -> Bus Creator/12  "ESP_ESPFunctionStatus"
  GW_3A1/13(ESP_EBDFailStatus_Out) -> Bus Creator/13  "ESP_EBDFailStatus"
  GW_3A1/14(EPS_EPSFailed_Out) -> Bus Creator/14  "EPS_EPSFailed"
  GW_3A1/15(EPB_FunctionLamp_Out) -> Bus Creator/15  "EPB_FunctionLamp"
  GW_3A1/16(EPB_SwitchPosition_Out) -> Bus Creator/16  "EPB_SwitchPosition"
  GW_3A1/17(EPB_SwitchPositionValid_Out) -> Bus Creator/17  "EPB_SwitchPositionValid"
  GW_3A1/18(ESP_HDC_STATUS_Out) -> Bus Creator/18  "ESP_HDC_STATUS"
  GW_3A1/19(ESP_AutoHoldAvailable_Out) -> Bus Creator/19  "ESP_AutoHoldAvailable"
  GW_3A1/20(ESP_HHC_Active_Out) -> Bus Creator/20  "ESP_HHC_Active"
  GW_3A1/21(ESP_AutoHoldActive_Out) -> Bus Creator/21  "ESP_AutoHoldActive"
  GW_3A1/22(ESP_HHC_Available_Out) -> Bus Creator/22  "ESP_HHC_Available"
  GW_3A1/23(TCU_GearForDisplay_Out) -> Bus Creator/23  "TCU_GearForDisplay"
  GW_3A1/24(ESP_HBBFunctionStatus_Out) -> Bus Creator/24  "ESP_HBBFunctionStatus"
  GW_3A1/25(TCU_GearIndication_Out) -> Bus Creator/25  "TCU_GearIndication"
  GW_3A1/26(TCU_ReqTranTempWarning_Out) -> Bus Creator/26  "TCU_ReqTranTempWarning"
  GW_3A1/27(EMS_RemindShiftGear_Out) -> Bus Creator/27  "EMS_RemindShiftGear"
  Signal Conversion/1 -> GW_3A2/1

== system VCU_CS75_12_27_test/长安CS75底盘程序，20ms一次/Input/CAN1_Rx/GW_567/ReceiveMessages/Subsystem ==
  input : Inport
  Enable : EnablePort
  Bus Creator : BusCreator  Inputs=5
  GW_2 : Subsystem
  Signal Conversion : SignalConversion
  GW_567 : Outport
  wires:
  Bus Creator/1 -> Signal Conversion/1
  input/1 -> GW_2/1(input)
  GW_2/1(HU_EnterTunnelInfo_Out) -> Bus Creator/1  "HU_EnterTunnelInfo"
  GW_2/2(HU_TunnelDistance_Out) -> Bus Creator/2  "HU_TunnelDistance"
  GW_2/3(HU_TunnelLength_Out) -> Bus Creator/3  "HU_TunnelLength"
  GW_2/4(HU_Byroad_Out) -> Bus Creator/4  "HU_Byroad"
  GW_2/5(HU_NavGuiganceStatus_Out) -> Bus Creator/5  "HU_NavGuiganceStatus"
  Signal Conversion/1 -> GW_567/1

== system VCU_CS75_12_27_test/长安CS75底盘程序，20ms一次/Input/CAN1_Rx/HU_GPS_500/ReceiveMessages/Subsystem ==
  input : Inport
  Enable : EnablePort
  Bus Creator : BusCreator  Inputs=1
  HU_GPS_1 : Subsystem
  Signal Conversion : SignalConversion
  HU_GPS_500 : Outport
  wires:
  input/1 -> HU_GPS_1/1(input)
  Bus Creator/1 -> Signal Conversion/1
  HU_GPS_1/1(GPSCurrentLocationValid_Out) -> Bus Creator/1  "GPSCurrentLocationValid"
  Signal Conversion/1 -> HU_GPS_500/1

== system VCU_CS75_12_27_test/长安CS75底盘程序，20ms一次/Input/CAN1_Rx/LAS_36E/ReceiveMessages/Subsystem ==
  input : Inport
  Enable : EnablePort
  Bus Creator : BusCreator  Inputs=7
  LAS_36E2 : Subsystem
  Signal Conversion : SignalConversion
  LAS_36E : Outport
  wires:
  Bus Creator/1 -> Signal Conversion/1
  input/1 -> LAS_36E2/1(input)
  LAS_36E2/1(LAS_RoadCurvatureFar_Out) -> Bus Creator/1  "LAS_RoadCurvatureFar"
  LAS_36E2/2(LAS_RoadCurvatureNear_Out) -> Bus Creator/2  "LAS_RoadCurvatureNear"
  LAS_36E2/3(LAS_LaneEquationC1_Out) -> Bus Creator/3  "LAS_LaneEquationC1"
  LAS_36E2/4(LAS_LaneEquationC3_Out) -> Bus Creator/4  "LAS_LaneEquationC3"
  LAS_36E2/5(LAS_RollingCounter_id36E_Out) -> Bus Creator/5  "LAS_RollingCounter_id36E"
  LAS_36E2/6(LAS_LaneEquationStatus_Out) -> Bus Creator/6  "LAS_LaneEquationStatus"
  LAS_36E2/7(LAS_CheckSum_id36E_Out) -> Bus Creator/7  "LAS_CheckSum_id36E"
  Signal Conversion/1 -> LAS_36E/1

== system VCU_CS75_12_27_test/长安CS75底盘程序，20ms一次/Input/CAN1_Rx/SAS_108/ReceiveMessages/Subsystem ==
  input : Inport
  Enable : EnablePort
  Bus Creator : BusCreator  Inputs=7
  SAS_2 : Subsystem
  Signal Conversion : SignalConversion
  SAS_108 : Outport
  wires:
  Bus Creator/1 -> Signal Conversion/1
  input/1 -> SAS_2/1(input)
  SAS_2/1(SAS_SteeringAngle_Out) -> Bus Creator/1  "SAS_SteeringAngle"
  SAS_2/2(SAS_SteeringAngleSpeed_Out) -> Bus Creator/2  "SAS_SteeringAngleSpeed"
  SAS_2/3(SAS_Calibrated_Out) -> Bus Creator/3  "SAS_Calibrated"
  SAS_2/4(SAS_SASFailure_Out) -> Bus Creator/4  "SAS_SASFailure"
  SAS_2/5(SAS_SteeringAngleValid_Out) -> Bus Creator/5  "SAS_SteeringAngleValid"
  SAS_2/6(SAS_RollingCounter_Out) -> Bus Creator/6  "SAS_RollingCounter"
  SAS_2/7(SAS_CRCCheck_Out) -> Bus Creator/7  "SAS_CRCCheck"
  Signal Conversion/1 -> SAS_108/1

== system VCU_CS75_12_27_test/长安CS75底盘程序，20ms一次/Input/CAN1_Rx/SCM_3B8/ReceiveMessages/Subsystem ==
  input : Inport
  Enable : EnablePort
  Bus Creator : BusCreator  Inputs=6
  SCM_3B2 : Subsystem
  Signal Conversion : SignalConversion
  SCM_3B8 : Outport
  wires:
  input/1 -> SCM_3B2/1(input)
  Bus Creator/1 -> Signal Conversion/1
  SCM_3B2/6(SCM_IACCOn_Out) -> Bus Creator/6  "SCM_IACCOn"
  SCM_3B2/5(SCM_TimeGap_Out) -> Bus Creator/5  "SCM_TimeGap"
  SCM_3B2/4(SCM_Speeddecrease_Out) -> Bus Creator/4  "SCM_Speeddecrease"
  SCM_3B2/3(SCM_Resume_Out) -> Bus Creator/3  "SCM_Resume"
  SCM_3B2/2(SCM_ACCCancel_Out) -> Bus Creator/2  "SCM_ACCCancel"
  SCM_3B2/1(SCM_ACCOn_Out) -> Bus Creator/1  "SCM_ACCOn"
  Signal Conversion/1 -> SCM_3B8/1

== system VCU_CS75_12_27_test/长安CS75底盘程序，20ms一次/Input/CAN1_Rx/SRS_005/ReceiveMessages/Subsystem ==
  input : Inport
  Enable : EnablePort
  Bus Creator : BusCreator  Inputs=2
  SRS_1 : Subsystem
  Signal Conversion : SignalConversion
  SRS_005 : Outport
  wires:
  Bus Creator/1 -> Signal Conversion/1
  input/1 -> SRS_1/1(input)
  SRS_1/1(SRS_DriverBuckleSwitchStatus_Out) -> Bus Creator/1  "SRS_DriverBuckleSwitchStatus"
  SRS_1/2(SRS_RollingCounter_Out) -> Bus Creator/2  "SRS_RollingCounter"
  Signal Conversion/1 -> SRS_005/1

== system VCU_CS75_12_27_test/长安CS75底盘程序，20ms一次/Input/CAN1_Rx/TCU_286/ReceiveMessages/Subsystem ==
  input : Inport
  Enable : EnablePort
  Bus Creator : BusCreator
  Signal Conversion : SignalConversion
  TCU_1 : Subsystem
  TCU_286 : Outport
  wires:
  input/1 -> TCU_1/1(input)
  Bus Creator/1 -> Signal Conversion/1
  TCU_1/1(TCU_ActualGear_Out) -> Bus Creator/1  "TCU_ActualGear"
  TCU_1/2(TCU_ShiftPositionValid_Out) -> Bus Creator/2  "TCU_ShiftPositionValid"
  TCU_1/3(TCU_ActualGearValid_Out) -> Bus Creator/3  "TCU_ActualGearValid"
  TCU_1/4(TCU_GearShiftPosition_Out) -> Bus Creator/4  "TCU_GearShiftPosition"
  Signal Conversion/1 -> TCU_286/1

== system VCU_CS75_12_27_test/长安CS75底盘程序，20ms一次/Input/DBC转化的messages（存底）/ReceiveMessages/EMS_205/EMS_CheckSum_205_Sub ==
  In1 : Inport
  Out1 : Outport
  wires:
  In1/1 -> Out1/1

== system VCU_CS75_12_27_test/长安CS75底盘程序，20ms一次/Input/DBC转化的messages（存底）/ReceiveMessages/EMS_205/EMS_ESPTorqReuestAvailability_Sub ==
  In1 : Inport
  Out1 : Outport
  wires:
  In1/1 -> Out1/1

== system VCU_CS75_12_27_test/长安CS75底盘程序，20ms一次/Input/DBC转化的messages（存底）/ReceiveMessages/EMS_205/EMS_FrictionalTorq_Sub ==
  In1 : Inport
  Out1 : Outport
  wires:
  In1/1 -> Out1/1

== system VCU_CS75_12_27_test/长安CS75底盘程序，20ms一次/Input/DBC转化的messages（存底）/ReceiveMessages/EMS_205/EMS_IndicatedDriverReqTorq_Sub ==
  In1 : Inport
  Out1 : Outport
  wires:
  In1/1 -> Out1/1

== system VCU_CS75_12_27_test/长安CS75底盘程序，20ms一次/Input/DBC转化的messages（存底）/ReceiveMessages/EMS_205/EMS_IndicatedRealEngTorq_Sub ==
  In1 : Inport
  Out1 : Outport
  wires:
  In1/1 -> Out1/1

== system VCU_CS75_12_27_test/长安CS75底盘程序，20ms一次/Input/DBC转化的messages（存底）/ReceiveMessages/EMS_205/EMS_RollingCounter_id205_Sub ==
  In1 : Inport
  Out1 : Outport
  wires:
  In1/1 -> Out1/1

== system VCU_CS75_12_27_test/长安CS75底盘程序，20ms一次/Input/DBC转化的messages（存底）/ReceiveMessages/EMS_205/EMS_TorqFailure_Sub ==
  In1 : Inport
  Out1 : Outport
  wires:
  In1/1 -> Out1/1

== system VCU_CS75_12_27_test/长安CS75底盘程序，20ms一次/Input/DBC转化的messages（存底）/ReceiveMessages1/EMS_255/EMS_AccPedal_Sub ==
  In1 : Inport
  Out1 : Outport
  wires:
  In1/1 -> Out1/1

== system VCU_CS75_12_27_test/长安CS75底盘程序，20ms一次/Input/DBC转化的messages（存底）/ReceiveMessages1/EMS_255/EMS_AccpedelError_Sub ==
  In1 : Inport
  Out1 : Outport
  wires:
  In1/1 -> Out1/1

== system VCU_CS75_12_27_test/长安CS75底盘程序，20ms一次/Input/DBC转化的messages（存底）/ReceiveMessages1/EMS_255/EMS_BrakePedalStatus_Sub ==
  In1 : Inport
  Out1 : Outport
  wires:
  In1/1 -> Out1/1

== system VCU_CS75_12_27_test/长安CS75底盘程序，20ms一次/Input/DBC转化的messages（存底）/ReceiveMessages1/EMS_255/EMS_CheckSum_255_Sub ==
  In1 : Inport
  Out1 : Outport
  wires:
  In1/1 -> Out1/1

== system VCU_CS75_12_27_test/长安CS75底盘程序，20ms一次/Input/DBC转化的messages（存底）/ReceiveMessages1/EMS_255/EMS_EngineSpeedError_Sub ==
  In1 : Inport
  Out1 : Outport
  wires:
  In1/1 -> Out1/1

== system VCU_CS75_12_27_test/长安CS75底盘程序，20ms一次/Input/DBC转化的messages（存底）/ReceiveMessages1/EMS_255/EMS_EngineSpeed_Sub ==
  In1 : Inport
  Out1 : Outport
  wires:
  In1/1 -> Out1/1

== system VCU_CS75_12_27_test/长安CS75底盘程序，20ms一次/Input/DBC转化的messages（存底）/ReceiveMessages1/EMS_255/EMS_RollingCounter_id255_Sub ==
  In1 : Inport
  Out1 : Outport
  wires:
  In1/1 -> Out1/1

== system VCU_CS75_12_27_test/长安CS75底盘程序，20ms一次/Input/DBC转化的messages（存底）/ReceiveMessages10/ESP_287/ESP_CheckSum_Sub ==
  In1 : Inport
  Out1 : Outport
  wires:
  In1/1 -> Out1/1

== system VCU_CS75_12_27_test/长安CS75底盘程序，20ms一次/Input/DBC转化的messages（存底）/ReceiveMessages10/ESP_287/ESP_HBBActiveStatus_Sub ==
  In1 : Inport
  Out1 : Outport
  wires:
  In1/1 -> Out1/1

== system VCU_CS75_12_27_test/长安CS75底盘程序，20ms一次/Input/DBC转化的messages（存底）/ReceiveMessages10/ESP_287/ESP_HBB_Status_Sub ==
  In1 : Inport
  Out1 : Outport
  wires:
  In1/1 -> Out1/1

== system VCU_CS75_12_27_test/长安CS75底盘程序，20ms一次/Input/DBC转化的messages（存底）/ReceiveMessages10/ESP_287/ESP_HDC_Status_Sub ==
  In1 : Inport
  Out1 : Outport
  wires:
  In1/1 -> Out1/1

== system VCU_CS75_12_27_test/长安CS75底盘程序，20ms一次/Input/DBC转化的messages（存底）/ReceiveMessages10/ESP_287/ESP_HHC_Available_Sub ==
  In1 : Inport
  Out1 : Outport
  wires:
  In1/1 -> Out1/1

== system VCU_CS75_12_27_test/长安CS75底盘程序，20ms一次/Input/DBC转化的messages（存底）/ReceiveMessages10/ESP_287/ESP_LatAcceleration_Sub ==
  In1 : Inport
  Out1 : Outport
  wires:
  In1/1 -> Out1/1

== system VCU_CS75_12_27_test/长安CS75底盘程序，20ms一次/Input/DBC转化的messages（存底）/ReceiveMessages10/ESP_287/ESP_LongAccelValid_Sub ==
  In1 : Inport
  Out1 : Outport
  wires:
  In1/1 -> Out1/1

== system VCU_CS75_12_27_test/长安CS75底盘程序，20ms一次/Input/DBC转化的messages（存底）/ReceiveMessages10/ESP_287/ESP_LongAcceleration_Sub ==
  In1 : Inport
  Out1 : Outport
  wires:
  In1/1 -> Out1/1

== system VCU_CS75_12_27_test/长安CS75底盘程序，20ms一次/Input/DBC转化的messages（存底）/ReceiveMessages10/ESP_287/ESP_RollingCounter_Sub ==
  In1 : Inport
  Out1 : Outport
  wires:
  In1/1 -> Out1/1

== system VCU_CS75_12_27_test/长安CS75底盘程序，20ms一次/Input/DBC转化的messages（存底）/ReceiveMessages10/ESP_287/ESP_TODFastOpenRequest_Sub ==
  In1 : Inport
  Out1 : Outport
  wires:
  In1/1 -> Out1/1

== system VCU_CS75_12_27_test/长安CS75底盘程序，20ms一次/Input/DBC转化的messages（存底）/ReceiveMessages10/ESP_287/ESP_TODTorqueMaxLimit_Sub ==
  In1 : Inport
  Out1 : Outport
  wires:
  In1/1 -> Out1/1

== system VCU_CS75_12_27_test/长安CS75底盘程序，20ms一次/Input/DBC转化的messages（存底）/ReceiveMessages10/ESP_287/ESP_YawRate_Status_Sub ==
  In1 : Inport
  Out1 : Outport
  wires:
  In1/1 -> Out1/1

== system VCU_CS75_12_27_test/长安CS75底盘程序，20ms一次/Input/DBC转化的messages（存底）/ReceiveMessages10/ESP_287/ESP_YawRate_Sub ==
  In1 : Inport
  Out1 : Outport
  wires:
  In1/1 -> Out1/1

== system VCU_CS75_12_27_test/长安CS75底盘程序，20ms一次/Input/DBC转化的messages（存底）/ReceiveMessages11/HU_AEBSetting_551/HU_AEBOnOffSetting_Sub ==
  In1 : Inport
  Out1 : Outport
  wires:
  In1/1 -> Out1/1

== system VCU_CS75_12_27_test/长安CS75底盘程序，20ms一次/Input/DBC转化的messages（存底）/ReceiveMessages11/HU_AEBSetting_551/HU_FCWSetting_Sub ==
  In1 : Inport
  Out1 : Outport
  wires:
  In1/1 -> Out1/1

== system VCU_CS75_12_27_test/长安CS75底盘程序，20ms一次/Input/DBC转化的messages（存底）/ReceiveMessages11/HU_AEBSetting_551/HU_LCASetting_Sub ==
  In1 : Inport
  Out1 : Outport
  wires:
  In1/1 -> Out1/1

== system VCU_CS75_12_27_test/长安CS75底盘程序，20ms一次/Input/DBC转化的messages（存底）/ReceiveMessages12/HU_LASSetting_0x541/HU_AudioWarningEnable_Sub ==
  In1 : Inport
  Out1 : Outport
  wires:
  In1/1 -> Out1/1

== system VCU_CS75_12_27_test/长安CS75底盘程序，20ms一次/Input/DBC转化的messages（存底）/ReceiveMessages12/HU_LASSetting_0x541/HU_BSD_LCAEnable_Sub ==
  In1 : Inport
  Out1 : Outport
  wires:
  In1/1 -> Out1/1

== system VCU_CS75_12_27_test/长安CS75底盘程序，20ms一次/Input/DBC转化的messages（存底）/ReceiveMessages12/HU_LASSetting_0x541/HU_CTAEnable_Sub ==
  In1 : Inport
  Out1 : Outport
  wires:
  In1/1 -> Out1/1

== system VCU_CS75_12_27_test/长安CS75底盘程序，20ms一次/Input/DBC转化的messages（存底）/ReceiveMessages12/HU_LASSetting_0x541/HU_DSMMemoryPositionFeedback_Sub ==
  In1 : Inport
  Out1 : Outport
  wires:
  In1/1 -> Out1/1

== system VCU_CS75_12_27_test/长安CS75底盘程序，20ms一次/Input/DBC转化的messages（存底）/ReceiveMessages12/HU_LASSetting_0x541/HU_DVRBrowseCommand_Sub ==
  In1 : Inport
  Out1 : Outport
  wires:
  In1/1 -> Out1/1

== system VCU_CS75_12_27_test/长安CS75底盘程序，20ms一次/Input/DBC转化的messages（存底）/ReceiveMessages12/HU_LASSetting_0x541/HU_HMAEnable_Sub ==
  In1 : Inport
  Out1 : Outport
  wires:
  In1/1 -> Out1/1

== system VCU_CS75_12_27_test/长安CS75底盘程序，20ms一次/Input/DBC转化的messages（存底）/ReceiveMessages12/HU_LASSetting_0x541/HU_IACCEnable_Sub ==
  In1 : Inport
  Out1 : Outport
  wires:
  In1/1 -> Out1/1

== system VCU_CS75_12_27_test/长安CS75底盘程序，20ms一次/Input/DBC转化的messages（存底）/ReceiveMessages12/HU_LASSetting_0x541/HU_LASModeSelection_Sub ==
  In1 : Inport
  Out1 : Outport
  wires:
  In1/1 -> Out1/1
